simulink model "Non_Linear_Simulator_Jetstar"  (R2020a)
settings: Solver=ode4  StartTime=0.0  StopTime=200  FixedStep=0.01  RelTol=1e-3
model workspace: external: MAT-File E:\Autopilot\Task 7\GP04_Task7_Codes\JETSTAR_FC4_Parameters.mat (data not in the file)
values from neighbouring files (symbols this model uses):
  g = 32.17405    [JETSTAR_FC4_Parameters.mat]    (also in ReadExcelModified.m = aircraft_data(52))
  Ixx = 118779    [JETSTAR_FC4_Parameters.mat]    (also in ReadExcelModified.m = aircraft_data(53))
  Ixy = 0    [JETSTAR_FC4_Parameters.mat]    (also in ReadExcelModified.m)
  Ixz = 5061    [JETSTAR_FC4_Parameters.mat]    (also in ReadExcelModified.m = aircraft_data(56))
  Iyy = 135876    [JETSTAR_FC4_Parameters.mat]    (also in ReadExcelModified.m = aircraft_data(54))
  Iyz = 0    [JETSTAR_FC4_Parameters.mat]    (also in ReadExcelModified.m)
  Izz = 243513    [JETSTAR_FC4_Parameters.mat]    (also in ReadExcelModified.m = aircraft_data(55))
  m = 1187.44764803    [JETSTAR_FC4_Parameters.mat]    (also in ReadExcelModified.m = aircraft_data(51))
  p_0 = 0    [JETSTAR_FC4_Parameters.mat]    (also in ReadExcelModified.m = s0(4))
  phi_0 = 0    [JETSTAR_FC4_Parameters.mat]    (also in ReadExcelModified.m = s0(7))
  psi_0 = 0    [JETSTAR_FC4_Parameters.mat]    (also in ReadExcelModified.m = s0(9))
  q_0 = 0    [JETSTAR_FC4_Parameters.mat]    (also in ReadExcelModified.m = s0(5))
  r_0 = 0    [JETSTAR_FC4_Parameters.mat]    (also in ReadExcelModified.m = s0(6))
  theta_0 = 0.0471238898038    [JETSTAR_FC4_Parameters.mat]    (also in ReadExcelModified.m = s0(8))
  u_0 = 585.349466728    [JETSTAR_FC4_Parameters.mat]    (also in ReadExcelModified.m = s0(1))
  v_0 = 0    [JETSTAR_FC4_Parameters.mat]    (also in ReadExcelModified.m = s0(2))
  w_0 = 27.6043801159    [JETSTAR_FC4_Parameters.mat]    (also in ReadExcelModified.m = s0(3))
  wdot_0 = 0    [JETSTAR_FC4_Parameters.mat]    (also in ReadExcelModified.m)
  x_0 = 0    [JETSTAR_FC4_Parameters.mat]    (also in ReadExcelModified.m = s0(10))
  y_0 = 0    [JETSTAR_FC4_Parameters.mat]    (also in ReadExcelModified.m = s0(11))
  z_0 = 0    [JETSTAR_FC4_Parameters.mat]    (also in ReadExcelModified.m = s0(12))
libraries: shared6dof x1, aerolibasang x1
settings Model: OrderedModelArguments=off  Creator=mohan  LastModifiedBy=mohan
settings SolverCC: AlgebraicLoopSolver=LineSearch

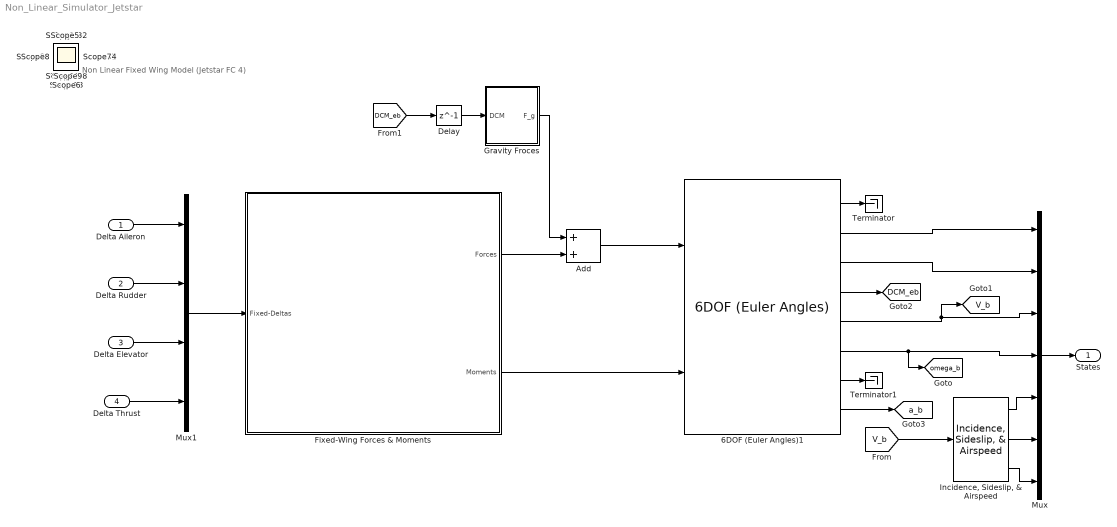
== system Non_Linear_Simulator_Jetstar ==
  note: Non Linear Fixed Wing Model (Jetstar FC 4)
  Delta Aileron : Inport
  Delta Rudder : Inport  Port=2
  Delta Elevator : Inport  Port=3
  Delta Thrust : Inport  Port=4
  6DOF (Euler Angles)1 : shared6dof/6DOF (Euler Angles)  units=English (Velocity in ft/s)  mtype=Fixed  rep=Euler Angles  xme_0=[x_0 y_0 z_0]  Vm_0=[u_0 v_0 w_0]  eul_0=[phi_0 theta_0 psi_0]  pm_0=[p_0 q_0 r_0]  mass_0=m  mass_e=0.5  mass_f=2.0  inertia=[Ixx -Ixy -Ixz ; -Ixy Iyy -Iyz ; -Ixz -Iyz Izz]  inertia_e=eye(3)  inertia_f=2*eye(3)  k_quat=1.0  vre_flag=on  abi_flag=off  aMode=aMode  xme_statename=''  Vm_statename=''  eul_statename=''  quat_statename=''  pm_statename=''  mass_statename=''
      settings: SourceProductBaseCode=AE,PW,MT,VE,VP
  Add : Sum  Inputs=2
  Delay : Delay  DelayLength=1  InitialCondition="inv([cos(theta_0)*cos(psi_0) , (sin(phi_0)*sin(theta_0)*cos(psi_0)-cos(phi_0)*sin(psi_0)) , (cos(phi_0)*sin(theta_0)*cos(psi_0)+sin(phi_0)*sin(psi_0)) ; cos(theta_0)*sin(psi_0) , (sin(phi_0)*sin(theta_0)*sin(psi_0)+cos(phi_0)*cos(psi_0)) , (cos(phi_0)*sin(theta_0)*sin(psi_0)-sin(phi_0)*cos(psi_0)) ;  -sin(theta_0) ,  sin(phi_0)*cos(theta_0)  , cos(phi_0)*cos(theta_0)])"
  Fixed-Wing Forces & Moments : Subsystem
  Gravity Froces : Subsystem
  "Incidence, Sideslip, & Airspeed" : aerolibasang/Incidence, Sideslip, & Airspeed
  Mux : Mux  Inputs=7
  Mux1 : Mux
  Terminator : Terminator
  Terminator1 : Terminator
  States : Outport
  Scope{,1..35} (36 alike) : Scope
  tag scope: DCM_eb=global, V_b=global, a_b=global, omega_b=global
  wires:
  Delay/1 -> Gravity Froces/1(DCM)
  6DOF (Euler Angles)1/6 -> [omega_b], Mux/4
  6DOF (Euler Angles)1/5 -> [V_b], Mux/3
  6DOF (Euler Angles)1/3 -> Mux/2
  [DCM_eb] -> Delay/1
  6DOF (Euler Angles)1/8 -> [a_b]
  6DOF (Euler Angles)1/4 -> [DCM_eb]
  Fixed-Wing Forces & Moments/2("Moments ") -> 6DOF (Euler Angles)1/2
  Add/1 -> 6DOF (Euler Angles)1/1
  Fixed-Wing Forces & Moments/1(Forces) -> Add/2
  6DOF (Euler Angles)1/7 -> Terminator1/1
  Mux/1 -> States/1
  6DOF (Euler Angles)1/1 -> Terminator/1
  6DOF (Euler Angles)1/2 -> Mux/1
  Gravity Froces/1(F_g) -> Add/1
  Delta Thrust/1 -> Mux1/4
  Delta Aileron/1 -> Mux1/1
  Delta Elevator/1 -> Mux1/3
  Delta Rudder/1 -> Mux1/2
  Mux1/1 -> Fixed-Wing Forces & Moments/1(Fixed-Deltas)
  [V_b] -> "Incidence, Sideslip, & Airspeed"/1
  "Incidence, Sideslip, & Airspeed"/1 -> Mux/5
  "Incidence, Sideslip, & Airspeed"/2 -> Mux/6
  "Incidence, Sideslip, & Airspeed"/3 -> Mux/7

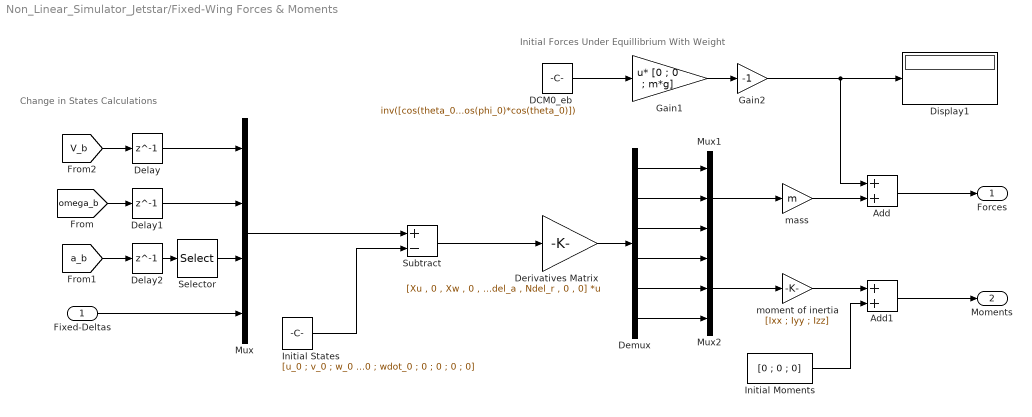
== system Non_Linear_Simulator_Jetstar/Fixed-Wing Forces & Moments ==
  note: Change in States Calculations
  note: Initial Forces Under Equillibrium With Weight
  Fixed-Deltas : Inport
  Add : Sum
  Add1 : Sum
  DCM0_eb : Constant  Value="inv([cos(theta_0)*cos(psi_0) , (sin(phi_0)*sin(theta_0)*cos(psi_0)-cos(phi_0)*sin(psi_0)) , (cos(phi_0)*sin(theta_0)*cos(psi_0)+sin(phi_0)*sin(psi_0)) ; cos(theta_0)*sin(psi_0) , (sin(phi_0)*sin(theta_0)*sin(psi_0)+cos(phi_0)*cos(psi_0)) , (cos(phi_0)*sin(theta_0)*sin(psi_0)-sin(phi_0)*cos(psi_0)) ;  -sin(theta_0) ,  sin(phi_0)*cos(theta_0)  , cos(phi_0)*cos(theta_0)])"
  Delay : Delay  DelayLength=1  InitialCondition=[u_0 v_0 w_0]
  Delay1 : Delay  DelayLength=1  InitialCondition=[p_0 q_0 r_0]
  Delay2 : Delay  DelayLength=1  InitialCondition=[0 0 wdot_0]
  Demux : Demux  Outputs=6
  Derivatives Matrix : Gain  Gain=[Xu , 0 , Xw , 0 , 0 , 0 , 0 , 0 , 0 , Xdel_e, Xdel_t ; 0 , Yv , 0 , 0 , 0 , 0 , 0 , 0 , Ydel_r , 0 , 0 ; Zu , 0 , Zw , 0 , Zq , 0 , Zw_dot , 0 , 0 , Zdel_e , Zdel_t ; 0 , Lv , 0 , Lp , 0 , Lr , 0 , Ldel_a , Ldel_r , 0 , 0 ; Mu , 0 , Mw , 0 , Mq , 0 , Mw_dot , 0 , 0 , Mdel_e , Mdel_t ; 0 , Nv , 0 , Np , 0 , Nr , 0 , Ndel_a , Ndel_r , 0 , 0]  Multiplication=Matrix(K*u)
  Display1 : Display
      settings: Decimation=4
  Gain1 : Gain  Gain=[0 ; 0 ; m*g]  Multiplication=Matrix(u*K)
  Gain2 : Gain  Gain=-1
  Initial Moments : Constant  Value=[0 ; 0 ; 0]
  Initial States : Constant  Value=[u_0 ; v_0 ; w_0 ; p_0 ; q_0 ; r_0 ; wdot_0 ; 0 ; 0 ; 0 ; 0]
  Mux : Mux
  Mux1 : Mux  Inputs=3
  Mux2 : Mux  Inputs=3
  Selector : Selector  InputPortWidth=3  IndexOptions=Starting index (dialog)  Indices=3  OutputSizes=1
  Subtract : Sum  Inputs=+-
  mass : Gain  Gain=m
  moment of inertia : Gain  Gain=[Ixx ; Iyy ; Izz]
  Forces : Outport
  "Moments " : Outport  Port=2
  wires:
  Fixed-Deltas/1 -> Mux/4
  [omega_b] -> Delay1/1
  [V_b] -> Delay/1
  Mux/1 -> Subtract/1
  Initial States/1 -> Subtract/2
  Demux/2 -> Mux1/2
  Demux/1 -> Mux1/1
  Demux/3 -> Mux1/3
  Demux/4 -> Mux2/1
  Demux/5 -> Mux2/2
  Demux/6 -> Mux2/3
  Mux1/1 -> mass/1
  Mux2/1 -> moment of inertia/1
  mass/1 -> Add/2
  moment of inertia/1 -> Add1/1
  Add/1 -> Forces/1
  Add1/1 -> "Moments "/1
  DCM0_eb/1 -> Gain1/1
  Gain1/1 -> Gain2/1
  Gain2/1 -> Add/1, Display1/1
  Initial Moments/1 -> Add1/2
  Derivatives Matrix/1 -> Demux/1
  [a_b] -> Delay2/1
  Delay/1 -> Mux/1
  Delay1/1 -> Mux/2
  Selector/1 -> Mux/3
  Delay2/1 -> Selector/1
  Subtract/1 -> Derivatives Matrix/1

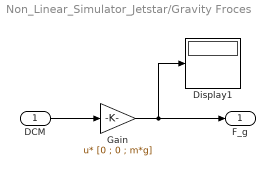
== system Non_Linear_Simulator_Jetstar/Gravity Froces ==
  DCM : Inport
  Display1 : Display
  Gain : Gain  Gain=[0 ; 0 ; m*g]  Multiplication=Matrix(u*K)
  F_g : Outport
  wires:
  Gain/1 -> F_g/1, Display1/1
  DCM/1 -> Gain/1
